simulink model "ilst_filter"  (R2021a)
settings: Solver=VariableStepAuto  StartTime=0.0  StopTime=10.0  RelTol=1e-3
libraries: spsSampleandHoldLib x3
settings Model: Creator=Dell  LastModifiedBy=Dell

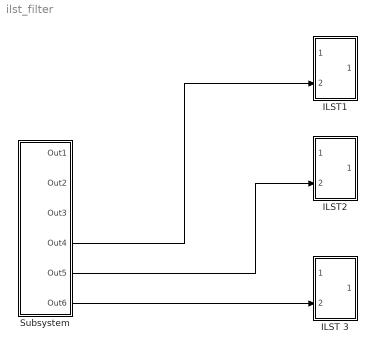
== system ilst_filter ==
  ILST 3 : Subsystem
  ILST1 : Subsystem
  ILST2 : Subsystem
  Subsystem : Subsystem
  wires:
  Subsystem/4(Out4) -> ILST1/2(In2)
  Subsystem/5(Out5) -> ILST2/2(In2)
  Subsystem/6(Out6) -> ILST 3/2(In2)

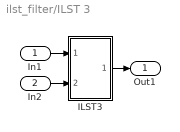
== system ilst_filter/ILST 3 ==
  In1 : Inport
  In2 : Inport  Port=2
  ILST3 : Subsystem
  Out1 : Outport
  wires:
  In1/1 -> ILST3/1(In1)
  In2/1 -> ILST3/2(In2)
  ILST3/1(Out1) -> Out1/1

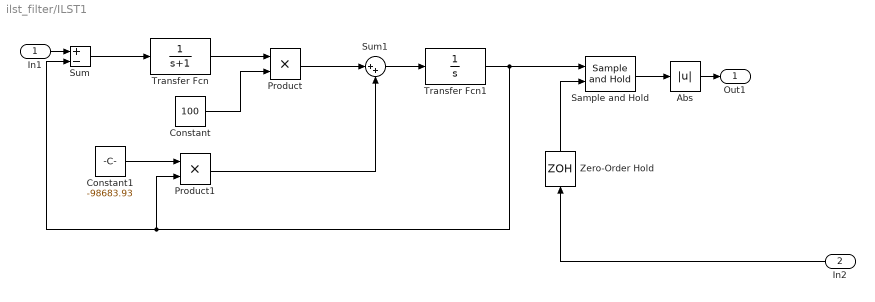
== system ilst_filter/ILST1 ==
  In1 : Inport
  In2 : Inport  Port=2
  Abs : Abs
  Constant : Constant  Value=100
  Constant1 : Constant  Value=-98683.93
  Product : Product
  Product1 : Product
  Sample and Hold : spsSampleandHoldLib/Sample and Hold  ic=0  Ts=0
      settings: SourceProductBaseCode=PS
  Sum : Sum  Inputs=+-
  Sum1 : Sum  Inputs=|++
  Transfer Fcn : TransferFcn  Denominator=[1 1]
  Transfer Fcn1 : TransferFcn  Denominator=[1 0]
  Zero-Order Hold : ZeroOrderHold  SampleTime=-1
  Out1 : Outport
  wires:
  Constant/1 -> Product/2
  Constant1/1 -> Product1/1
  Product/1 -> Sum1/1
  Zero-Order Hold/1 -> Sample and Hold/2
  Sum1/1 -> Transfer Fcn1/1
  In1/1 -> Sum/1
  Transfer Fcn1/1 -> Sample and Hold/1, Product1/2, Sum/2
  Product1/1 -> Sum1/2
  Transfer Fcn/1 -> Product/1
  Sum/1 -> Transfer Fcn/1
  Sample and Hold/1 -> Abs/1
  In2/1 -> Zero-Order Hold/1
  Abs/1 -> Out1/1

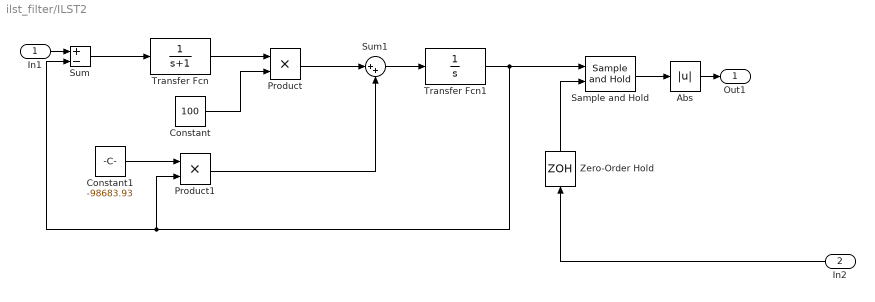
== system ilst_filter/ILST2 ==
  In1 : Inport
  In2 : Inport  Port=2
  Abs : Abs
  Constant : Constant  Value=100
  Constant1 : Constant  Value=-98683.93
  Product : Product
  Product1 : Product
  Sample and Hold : spsSampleandHoldLib/Sample and Hold  ic=0  Ts=0
      settings: SourceProductBaseCode=PS
  Sum : Sum  Inputs=+-
  Sum1 : Sum  Inputs=|++
  Transfer Fcn : TransferFcn  Denominator=[1 1]
  Transfer Fcn1 : TransferFcn  Denominator=[1 0]
  Zero-Order Hold : ZeroOrderHold  SampleTime=-1
  Out1 : Outport
  wires:
  Constant/1 -> Product/2
  Constant1/1 -> Product1/1
  Product/1 -> Sum1/1
  Zero-Order Hold/1 -> Sample and Hold/2
  Sum1/1 -> Transfer Fcn1/1
  In1/1 -> Sum/1
  Transfer Fcn1/1 -> Sample and Hold/1, Product1/2, Sum/2
  Product1/1 -> Sum1/2
  Transfer Fcn/1 -> Product/1
  Sum/1 -> Transfer Fcn/1
  Sample and Hold/1 -> Abs/1
  In2/1 -> Zero-Order Hold/1
  Abs/1 -> Out1/1

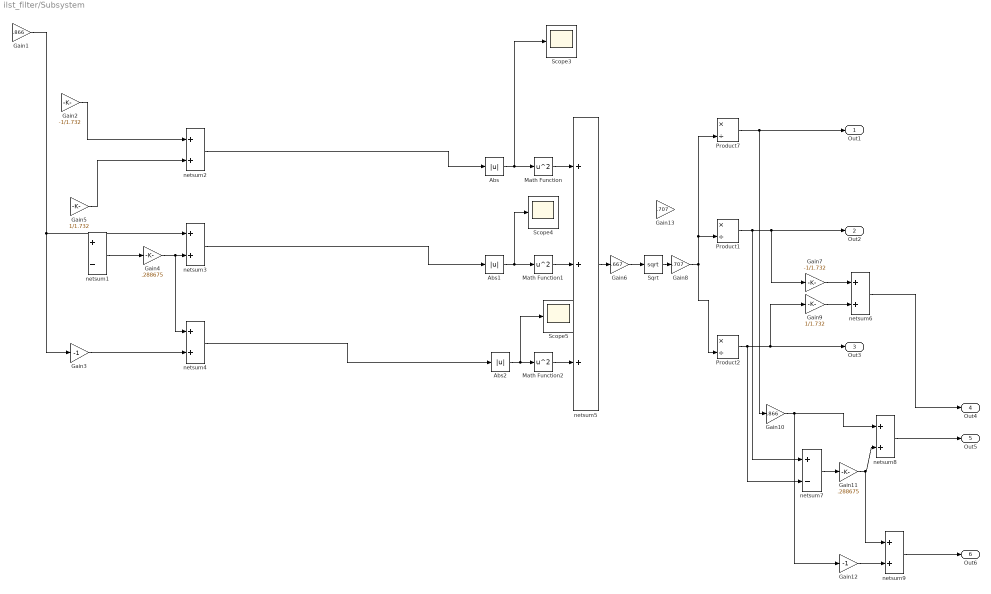
== system ilst_filter/Subsystem ==
  Abs : Abs
  Abs1 : Abs
  Abs2 : Abs
  Gain1 : Gain  Gain=.866
  Gain10 : Gain  Gain=.866
  Gain11 : Gain  Gain=.288675
  Gain12 : Gain  Gain=-1
  Gain13 : Gain  Gain=.707
  Gain2 : Gain  Gain=-1/1.732
  Gain3 : Gain  Gain=-1
  Gain4 : Gain  Gain=.288675
  Gain5 : Gain  Gain=1/1.732
  Gain6 : Gain  Gain=.667
  Gain7 : Gain  Gain=-1/1.732
  Gain8 : Gain  Gain=.707
  Gain9 : Gain  Gain=1/1.732
  Math Function : Math  Operator=square  SignedPower=on  SaturateOnIntegerOverflow=on
  Math Function1 : Math  Operator=square  SignedPower=on  SaturateOnIntegerOverflow=on
  Math Function2 : Math  Operator=square  SignedPower=on  SaturateOnIntegerOverflow=on
  Product1 : Product  Inputs=*/  RndMeth=Zero
  Product2 : Product  Inputs=*/  RndMeth=Zero
  Product7 : Product  Inputs=*/  RndMeth=Zero
  Scope3 : Scope
  Scope4 : Scope
  Scope5 : Scope
  Sqrt : Sqrt  SaturateOnIntegerOverflow=on
  netsum1 : Sum  Inputs=+-  InputSameDT=on  SaturateOnIntegerOverflow=on  OutDataTypeStr=Inherit: Same as first input
  netsum{2..4,6,8..9} (6 alike) : Sum  InputSameDT=on  SaturateOnIntegerOverflow=on  OutDataTypeStr=Inherit: Same as first input
  netsum5 : Sum  Inputs=+++  InputSameDT=on  SaturateOnIntegerOverflow=on  OutDataTypeStr=Inherit: Same as first input
  netsum7 : Sum  Inputs=+-  InputSameDT=on  SaturateOnIntegerOverflow=on  OutDataTypeStr=Inherit: Same as first input
  Out1 : Outport
  Out2 : Outport  Port=2
  Out3 : Outport  Port=3
  Out4 : Outport  Port=4
  Out5 : Outport  Port=5
  Out6 : Outport  Port=6
  wires:
  ? -> Product2/1, netsum1/2, Gain5/1
  ? -> netsum1/1, Product1/1, Gain2/1
  Gain9/1 -> netsum6/2
  Gain8/1 -> Product2/2, Product7/2, Product1/2
  Gain12/1 -> netsum9/2
  netsum2/1 -> Abs/1
  netsum9/1 -> Out6/1
  Gain3/1 -> netsum4/2
  netsum7/1 -> Gain11/1
  Gain4/1 -> netsum4/1, netsum3/2
  Gain5/1 -> netsum2/2
  netsum1/1 -> Gain4/1
  Math Function2/1 -> netsum5/3
  Gain1/1 -> Gain3/1, netsum3/1
  netsum8/1 -> Out5/1
  Product7/1 -> Gain10/1, Out1/1
  Gain2/1 -> netsum2/1
  Product2/1 -> netsum7/2, Gain9/1, Out3/1
  Math Function/1 -> netsum5/1
  ? -> Product7/1, Gain1/1
  Product1/1 -> netsum7/1, Out2/1, Gain7/1
  netsum3/1 -> Abs1/1
  Sqrt/1 -> Gain8/1
  Abs2/1 -> Scope5/1, Math Function2/1
  Gain11/1 -> netsum9/1, netsum8/2
  Abs1/1 -> Scope4/1, Math Function1/1
  netsum5/1 -> Gain6/1
  Gain6/1 -> Sqrt/1
  Math Function1/1 -> netsum5/2
  netsum4/1 -> Abs2/1
  Gain7/1 -> netsum6/1
  netsum6/1 -> Out4/1
  Gain10/1 -> Gain12/1, netsum8/1
  Abs/1 -> Scope3/1, Math Function/1

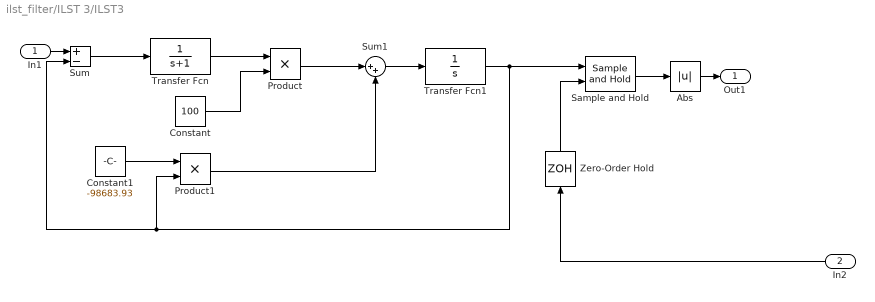
== system ilst_filter/ILST 3/ILST3 ==
  In1 : Inport
  In2 : Inport  Port=2
  Abs : Abs
  Constant : Constant  Value=100
  Constant1 : Constant  Value=-98683.93
  Product : Product
  Product1 : Product
  Sample and Hold : spsSampleandHoldLib/Sample and Hold  ic=0  Ts=0
      settings: SourceProductBaseCode=PS
  Sum : Sum  Inputs=+-
  Sum1 : Sum  Inputs=|++
  Transfer Fcn : TransferFcn  Denominator=[1 1]
  Transfer Fcn1 : TransferFcn  Denominator=[1 0]
  Zero-Order Hold : ZeroOrderHold  SampleTime=-1
  Out1 : Outport
  wires:
  Constant/1 -> Product/2
  Constant1/1 -> Product1/1
  Product/1 -> Sum1/1
  Zero-Order Hold/1 -> Sample and Hold/2
  Sum1/1 -> Transfer Fcn1/1
  In1/1 -> Sum/1
  Transfer Fcn1/1 -> Sample and Hold/1, Product1/2, Sum/2
  Product1/1 -> Sum1/2
  Transfer Fcn/1 -> Product/1
  Sum/1 -> Transfer Fcn/1
  Sample and Hold/1 -> Abs/1
  In2/1 -> Zero-Order Hold/1
  Abs/1 -> Out1/1
